simulink model "Load_Simulation_04"  (R2017a)
settings: Solver=ode23tb  StartTime=0.0  StopTime=3600  MaxStep=0.1  RelTol=1e-4  EnableMultiTasking=on
undefined symbols (not defined in the file or in its folder): Acid, Hydride, Ion, Lead, Lithium, Metal, Nickel, sigbuilder_block
libraries: powerlib x4, electricdrivelib x3
Description:
  | Copyright 2008-2017 The MathWorks, Inc.
settings Model: Creator=MathWorks  LastModifiedBy=hlope
settings DataIOCC: LimitDataPoints=on  SaveFormat=Array  SignalLoggingSaveFormat=ModelDataLogs
settings OptimizationCC: ExpressionDepthLimit=2147483647  InitFltsAndDblsToZero=on  LifeSpan=inf
settings DebuggingCC: UnderspecifiedInitializationDetection=Classic  MergeDetectMultiDrivingBlocksExec=none  SignalResolutionControl=TryResolveAllWithWarning  SolverPrmCheckMsg=warning  FcnCallInpInsideContextMsg=warning  AllowSymbolicDim=off  StateNameClashWarn=warning  SFUnexpectedBacktrackingDiag=warning  SFNoUnconditionalDefaultTransitionDiag=warning  SFExecutionAtInitializationDiag=none
settings HardwareCC: ProdBitPerPointer=32  ProdBitPerSizeT=32  ProdBitPerPtrDiffT=32  ProdLargestAtomicFloat=None  ProdIntDivRoundTo=Undefined  ProdEndianess=Unspecified  ProdWordSize=32  ProdHWDeviceType=32-bit Generic
settings ModelReferenceCC: PropagateSignalLabelsOutOfModel=off
settings GRTTargetCC: TargetLangStandard=C89/C90 (ANSI)  GeneratePreprocessorConditionals=Disable all  CombineOutputUpdateFcns=off  GRTInterface=on
settings ConfigComp: CovMetricSettings=dw  CovHtmlReporting=on  CovSaveCumulativeToWorkspaceVar=on  CovSaveSingleToWorkspaceVar=on  CovExternalEMLEnable=off

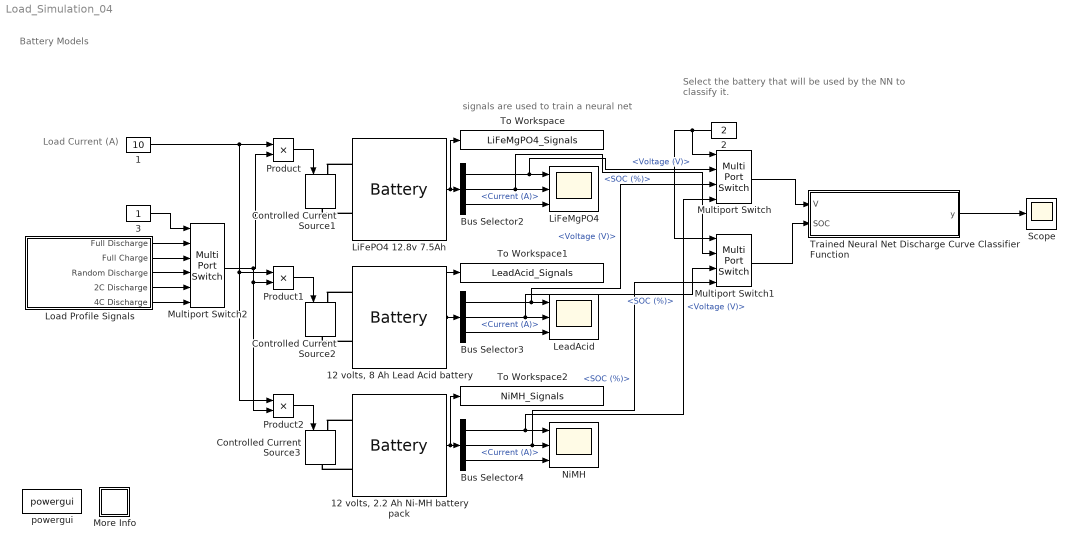
== system Load_Simulation_04 ==
  note: signals are used to train a neural net
  note: Select the battery that will be used by the NN
      | to classify it.
  note: Battery Models
  note: Load Current (A)
  " 1" : Constant  Value=10
  " 2" : Constant  Value=2
  " 3" : Constant
  "12 volts, 2.2 Ah Ni-MH battery pack" : electricdrivelib/Extra Sources/Battery  BatType=Nickel-Metal-Hydride  ShowTempParam=on  ThermalPreset=no  ShowAgeParam=off  NomV=12  NomQ=2.2  SOC=100  Batt_Tr=30  PresetModel=on  MaxQ=2.3692  MinV=9  FullV=14.1356  Dis_rate=0.44  R=0.054545  Normal_OP=2.1154  expZone="[13.0169         0.44]"  current=50  Units=Ampere-hour  Tci=20  NomT=25  T2=0  MaxQ2=2.208  FullV2=3.45  Normal_OP2=2.8  expZone2="[3.22        0.23]"  Rca=0.6  ti=1000  Dp=0  Neq0=0  Tsim=1e6  Ta1=25  Qeol=5.4*0.9  Reol=0.013333*1.2  Char_age=[2.3478, 3]  Dis_age=[2.3478, 10]  N1=1500  N2=10500  N3=1000  N4=1400  Ta2=45  N5=950
  "12 volts, 8 Ah Lead Acid battery " : electricdrivelib/Extra Sources/Battery  BatType=Lead-Acid  ShowTempParam=on  ThermalPreset=no  ShowAgeParam=off  NomV=12  NomQ=8  SOC=100  Batt_Tr=30  PresetModel=on  MaxQ=8.3333  MinV=9  FullV=13.0658  Dis_rate=1.6  R=0.015  Normal_OP=2.4822  expZone="[12.2171    0.0266667]"  current=50  Units=Ampere-hour  Tci=20  NomT=25  T2=0  MaxQ2=2.208  FullV2=3.45  Normal_OP2=2.8  expZone2="[3.22        0.23]"  Rca=0.6  ti=1000  Dp=0  Neq0=0  Tsim=1e6  Ta1=25  Qeol=5.4*0.9  Reol=0.013333*1.2  Char_age=[2.3478, 3]  Dis_age=[2.3478, 10]  N1=1500  N2=10500  N3=1000  N4=1400  Ta2=45  N5=950
  Bus Selector2 : BusSelector  OutputSignals=Voltage (V),SOC (%),Current (A)
  Bus Selector3 : BusSelector  OutputSignals=Voltage (V),SOC (%),Current (A)
  Bus Selector4 : BusSelector  OutputSignals=Voltage (V),SOC (%),Current (A)
  Controlled Current Source1 : powerlib/Electrical Sources/Controlled Current Source  Initialize=on  Source_Type=AC  Amplitude=0  Phase=0  Frequency=0  Measurements=None
  Controlled Current Source2 : powerlib/Electrical Sources/Controlled Current Source  Initialize=on  Source_Type=AC  Amplitude=0  Phase=0  Frequency=0  Measurements=None
  Controlled Current Source3 : powerlib/Electrical Sources/Controlled Current Source  Initialize=on  Source_Type=AC  Amplitude=0  Phase=0  Frequency=0  Measurements=None
  LeadAcid : Scope  NumInputPorts=3
  LiFeMgPO4 : Scope  NumInputPorts=3
  "LiFePO4 12.8v 7.5Ah " : electricdrivelib/Extra Sources/Battery  BatType=Lithium-Ion  ShowTempParam=off  ThermalPreset="12.8V  40Ah  (LiFeMgPO4)"  ShowAgeParam=off  NomV=12.8  NomQ=7.5  SOC=100  Batt_Tr=30  PresetModel=on  MaxQ=7.5  MinV=9.6  FullV=14.899  Dis_rate=3.2609  R=0.017067  Normal_OP=6.7826  expZone="[13.8289     0.368478]"  current=50  Units=Ampere-hour  Tci=20  NomT=20  T2=0  MaxQ2=36  FullV2=13  Normal_OP2=11.7  expZone2="[12.67            4]"  Rca=0.6411  ti=4880  Dp=0  Neq0=0  Tsim=1e6  Ta1=25  Qeol=5.4*0.9  Reol=0.013333*1.2  Char_age=[2.3478, 3]  Dis_age=[2.3478, 10]  N1=1500  N2=10500  N3=1000  N4=1400  Ta2=45  N5=950
  Load Profile Signals : Subsystem  Tag=STV Subsys  LoadFcn=sigbuilder_block('load');  StartFcn=sigbuilder_block('start');  StopFcn=sigbuilder_block('stop');  ClipboardFcn=sigbuilder_block('clipboard');  mask(Sigbuilder block){tuvar=[0:10]}
      mask help: Simulink:masks:SigbuilderBlock_MD
      mask init:
      | if ~strcmp(get_param(bdroot(gcbh),'SimulationStatus'),'stopped') tuvar = sigbuilder_block('maskInit'); end
      settings: CopyFcn=sigbuilder_block('copy');  DeleteFcn=sigbuilder_block('delete');  ModelCloseFcn=sigbuilder_block('modelClose');  PreSaveFcn=sigbuilder_block('preSave');  PauseFcn=sigbuilder_block('pause');  ContinueFcn=sigbuilder_block('continue');  NameChangeFcn=sigbuilder_block('namechange');  OpenFcn=sigbuilder_block('open',[243 30.6 574.8 516.6 ]);  CloseFcn=sigbuilder_block('close');
      mask Display: plot(0, 0, 100, 100,[2, 2, 32, 32, 2], [68, 8, 8, 68, 68],[32, 2], [38, 38], [32, 19, 2],[53, 60, 44], [32, 17, 17, 2],[16, 16, 31, 31]);txt = getActiveGroup(gcbh);text(2, 100, txt,'verticalAlignment', 'top');
  More Info : Subsystem
      settings: OpenFcn=showdemo(bdroot(gcb))
      mask Display: disp('?')
  Multiport Switch : MultiPortSwitch
  Multiport Switch1 : MultiPortSwitch
  Multiport Switch2 : MultiPortSwitch  Inputs=5
  NiMH : Scope  NumInputPorts=3
  Product : Product
  Product1 : Product
  Product2 : Product
  Scope : Scope
  To Workspace : ToWorkspace  VariableName=LiFeMgPO4_Signals  SaveFormat=Timeseries  SampleTime=-1
  To Workspace1 : ToWorkspace  VariableName=LeadAcid_Signals  SaveFormat=Timeseries  SampleTime=-1
  To Workspace2 : ToWorkspace  VariableName=NiMH_Signals  SaveFormat=Timeseries  SampleTime=-1
  Trained Neural Net Discharge Curve Classifier Function : MATLAB Function  TreatAsAtomicUnit=on
  powergui : powerlib/powergui  SimulationMode=Continuous  SampleTime=0.001  frequency=60  Iterations=50  frequencyindice=0  Pbase=100e6  ErrMax=1e-4  UnitsV=kV  UnitsW=MW  buscounter=0  FunctionMessages=off  echomessages=off  EnableUseOfTLC=off  CurrentSourceSwitches=off  DisableSnubberDevices=off  DisableRonSwitches=off  DisableVfSwitches=off  DisplayEquations=off  SolverType=Tustin  Interpol=off  ExternalGateDelay=off  methode=off  Ts=0  x0status=blocks  SPID=off  SwTol=0  HookPort=off  RestoreLinks=warning  ResistiveCurrentMeasurement=off  Frange=[0:2:500]  Ylog=off  Xlog=on  ShowGrid=off  save=off  variable=ZData  structure=0  ZoomFFT=on  StartTime=0.0  cycles=1  DisplayStyle=1  fundamental=60  FreqAxis=off  MaxFrequency=1000  frequencyindicesteady=1  RmsSteady=1  display=off
  wires:
  "12 volts, 2.2 Ah Ni-MH battery pack"/1 -> Bus Selector4/1, To Workspace2/1
  Bus Selector3/3 -> LeadAcid/3  "<Current (A)>"
  Bus Selector4/3 -> NiMH/3  "<Current (A)>"
  Bus Selector3/1 -> Multiport Switch/3, LeadAcid/1  "<Voltage (V)>"
  Product2/1 -> Controlled Current Source3/1
  "LiFePO4 12.8v 7.5Ah "/1 -> To Workspace/1, Bus Selector2/1
  Bus Selector3/2 -> LeadAcid/2, Multiport Switch1/3  "<SOC (%)>"
  Product1/1 -> Controlled Current Source2/1
  " 1"/1 -> Product/1, Product2/1, Product1/1
  Multiport Switch2/1 -> Product/2, Product2/2, Product1/2
  Bus Selector4/2 -> Multiport Switch1/4, NiMH/2  "<SOC (%)>"
  Bus Selector4/1 -> Multiport Switch/4, NiMH/1  "<Voltage (V)>"
  Bus Selector2/2 -> LiFeMgPO4/2, Multiport Switch1/2  "<SOC (%)>"
  Product/1 -> Controlled Current Source1/1
  Bus Selector2/1 -> Multiport Switch/2, LiFeMgPO4/1  "<Voltage (V)>"
  Bus Selector2/3 -> LiFeMgPO4/3  "<Current (A)>"
  "12 volts, 8 Ah Lead Acid battery "/1 -> To Workspace1/1, Bus Selector3/1
  Trained Neural Net Discharge Curve Classifier Function/1(y) -> Scope/1
  Multiport Switch/1 -> Trained Neural Net Discharge Curve Classifier Function/1(V)
  " 2"/1 -> Multiport Switch1/1, Multiport Switch/1
  Multiport Switch1/1 -> Trained Neural Net Discharge Curve Classifier Function/2(SOC)
  Load Profile Signals/3(Random Discharge) -> Multiport Switch2/4
  Load Profile Signals/2(Full Charge) -> Multiport Switch2/3
  Load Profile Signals/1(Full Discharge) -> Multiport Switch2/2
  Load Profile Signals/4(2C Discharge) -> Multiport Switch2/5
  Load Profile Signals/5(4C Discharge) -> Multiport Switch2/6
  " 3"/1 -> Multiport Switch2/1
  connections:
  "LiFePO4 12.8v 7.5Ah "/LConn2 -- Controlled Current Source1/RConn1
  "12 volts, 8 Ah Lead Acid battery "/LConn1 -- Controlled Current Source2/LConn1
  "12 volts, 2.2 Ah Ni-MH battery pack"/LConn2 -- Controlled Current Source3/RConn1
  "12 volts, 2.2 Ah Ni-MH battery pack"/LConn1 -- Controlled Current Source3/LConn1
  "12 volts, 8 Ah Lead Acid battery "/LConn2 -- Controlled Current Source2/RConn1
  "LiFePO4 12.8v 7.5Ah "/LConn1 -- Controlled Current Source1/LConn1

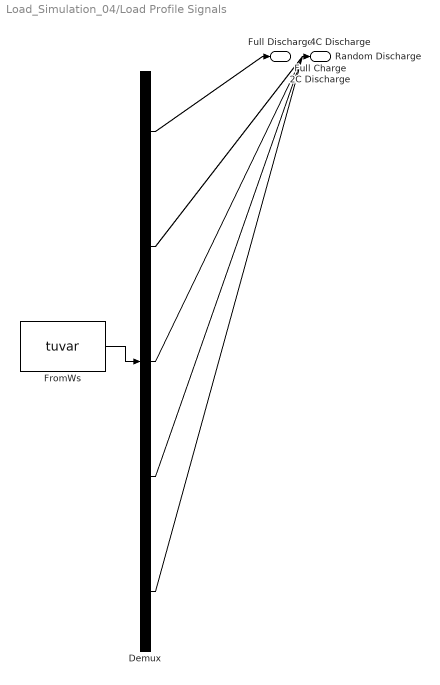
== system Load_Simulation_04/Load Profile Signals ==
  Demux : Demux  Tag=STV Demux  Outputs=5
  FromWs : FromWorkspace  Tag=STV FromWs  VariableName=tuvar  SampleTime=0
      SigBuilderData=|
      | common.afterFinalStr = 'Extrapolate'
      | common.sampleTime = 0
      | dataSet.timeRange = [0 3600]
      | dataSet.name = 'Load'
      | sbobj.Groups.Name = 'Load'
      | sbobj.Groups.Signals(1).Name = 'Full Discharge'
      | sbobj.Groups.Signals(1).XData = [0 1806 3502 3600]
      | sbobj.Groups.Signals(1).YData = [1 1 1 1]
      | sbobj.Groups.Signals(2).Name = 'Full Charge'
      | sbobj.Groups.Signals(2).XData = [0 3600]
      | sbobj.Groups.Signals(2).YData = [-0.98 -0.98]
      | sbobj.Groups.Signals(3).Name = 'Random Discharge'
      | sbobj.Groups.Signals(3).XData = [0 200 200 300 300 500 500 900 900 1000 1000 1100 1100 1500 1500 1900 1900 2200 2200 2500 2500 2600 2600 2700 2700 2800 2800 3000 3000 3100 3100 3500 3500 3600]
      | sbobj.Groups.Signals(3).YData = [0 0 1 1 0 0 1 1 0 0 1 1 0 0 1 1 0 0 1 1 0 0 1 1 0 0 1 1 0 0 1 1 0 0]
      | sbobj.Groups.Signals(4).Name = '2C Discharge'
      | sbobj.Groups.Signals(4).XData = [0 3600]
      | sbobj.Groups.Signals(4).YData = [0.5 0.5]
      | sbobj.Groups.Signals(5).Name = '4C Discharge'
      | sbobj.Groups.Signals(5).XData = [0 3600]
      | sbobj.Groups.Signals(5).YData = [0.25 0.25]
      | sbobj.Groups.TimeRange = [0 3600]
  Full Discharge : Outport  Tag=STV Outport
  Full Charge : Outport  Tag=STV Outport  Port=2
  Random Discharge : Outport  Tag=STV Outport  Port=3
  2C Discharge : Outport  Tag=STV Outport  Port=4
  4C Discharge : Outport  Tag=STV Outport  Port=5
  wires:
  FromWs/1 -> Demux/1
  Demux/1 -> Full Discharge/1
  Demux/2 -> Full Charge/1
  Demux/3 -> Random Discharge/1
  Demux/4 -> 2C Discharge/1
  Demux/5 -> 4C Discharge/1

== system Load_Simulation_04/More Info ==

== matlab function Load_Simulation_04/Trained Neural Net Discharge Curve Classifier Function ==
  data: V input; SOC input; y output
function y = fcn(V,SOC)

x1=[SOC,V];
o = Battery_Classifier(x1);
pcnt = mean(o.')';
[m,i]= max(pcnt);
y= i;
